simulink model "feux_signalisation"  (R2021a)
settings: Solver=FixedStepDiscrete  StartTime=0.0  StopTime=200  FixedStep=0.01  RelTol=1e-3
settings Model: Creator=Lenovo  LastModifiedBy=Lenovo
settings OptimizationCC: DefaultParameterBehavior=Inlined  EnhancedBackFolding=on  PassReuseOutputArgsAs=Individual arguments  ZeroExternalMemoryAtStartup=off  ZeroInternalMemoryAtStartup=off  OptimizeBlockOrder=speed  DifferentSizesBufferReuse=on  OptimizationCustomize=off  EfficientTunableParamExpr=on
settings DebuggingCC: ParameterTunabilityLossMsg=error
settings SFSimCC: MATLABDynamicMemAlloc=off
settings RTWCC: Description=AUTOSAR  SystemTargetFile=autosar.tlc  GenCodeOnly=on  TemplateMakefile=ert_default_tmf  CreateSILPILBlock=SIL
settings CodeAppCC: ForceParamTrailComments=on  IgnoreCustomStorageClasses=off  OperatorAnnotations=on  SimulinkDataObjDesc=on  SFDataObjDesc=on  InsertBlockDesc=on
settings STFCustomTargetCC: TargetLangStandard=C99 (ISO)  MultiwordLength=256  ParMdlRefBuildCompliant=on  CompOptLevelCompliant=on  IncludeMdlTerminateFcn=off  CombineOutputUpdateFcns=on  SuppressErrorStatus=on  ERTCustomFileBanners=on  SupportNonFinite=off  SupportComplex=off  SupportContinuousTime=off  SupportNonInlinedSFcns=off  RemoveResetFunc=on  MATLABClassNameForMDSCustomization=Simulink.SoftwareTarget.ERTCustomization  AutosarCompliant=on  GRTInterface=off  LookupTableObjectStructAxisOrder=2,1,3,4,...  LUTObjectStructOrderEvenSpacing=Size,Table,Breakpoints  SystemTargetFile=autosar.tlc
settings ERTTargetCC: TargetLangStandard=C99 (ISO)  ConcurrentExecutionCompliant=off  IncludeMdlTerminateFcn=off  SuppressErrorStatus=on  SupportNonFinite=off  SupportComplex=off  ModelStepFunctionPrototypeControlCompliant=off  CPPClassGenCompliant=off  AutosarCompliant=on  LookupTableObjectStructAxisOrder=2,1,3,4,...  LUTObjectStructOrderEvenSpacing=Size,Table,Breakpoints  InlinedParameterPlacement=NonHierarchical  ERTCustomFileTemplate=example_file_process.tlc

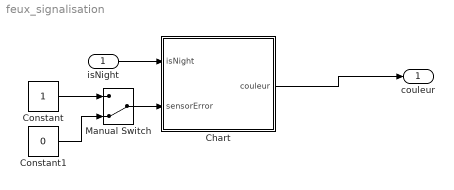
== system feux_signalisation ==
  isNight : Inport  OutDataTypeStr=boolean
  Chart : Stateflow chart  TreatAsAtomicUnit=on
  Constant : Constant  OutDataTypeStr=boolean
  Constant1 : Constant  Value=0  OutDataTypeStr=boolean
  Manual Switch : ManualSwitch  CurrentSetting=0
  couleur : Outport  SignalName=couleur
  wires:
  Chart/1(couleur) -> couleur/1
  isNight/1 -> Chart/1(isNight)
  Manual Switch/1 -> Chart/2(sensorError)
  Constant/1 -> Manual Switch/1
  Constant1/1 -> Manual Switch/2

== stateflow chart feux_signalisation/Chart ==
  state Mode_Degrade
    state Orange_Fast_ON
      entry:
      couleur = 2;
    state Orange_Fast_OFF
      entry:
      couleur = 0;
    (default) -> Orange_Fast_ON
    Orange_Fast_OFF -> Orange_Fast_ON : after(0.2, sec)
    Orange_Fast_ON -> Orange_Fast_OFF : after(0.2, sec)
  state Mode_nuit
    state Orange_ON
      entry:
      couleur = 2;
    state Orange_OFF
      entry:
      couleur = 0;
    (default) -> Orange_ON
    Orange_OFF -> Orange_ON : after(1, sec)
    Orange_ON -> Orange_OFF : after(1, sec)
  state Mode_Jour
    state vert
      entry:
      couleur = 1;
    state orange
      entry:
      couleur = 2;
    state rouge
      entry:
      couleur = 3;
    (default) -> vert
    rouge -> vert : after(30, sec)
    vert -> orange : after(30, sec)
    orange -> rouge : after(5, sec)
  Mode_nuit -> Mode_Degrade [order 1] : [sensorError == true]
  Mode_Jour -> Mode_Degrade [order 1] : [sensorError == true]
  (default) -> Mode_Jour
  Mode_Degrade -> Mode_Jour : [sensorError == false]
  Mode_Jour -> Mode_nuit [order 2] : [isNight == true]
  Mode_nuit -> Mode_Jour [order 2] : [isNight == false]
  data: isNight input boolean; sensorError input boolean; couleur output
